simulink model "lab2_sliding_mode_control"  (R2018b)
settings: Solver=ode1  StartTime=0.0  StopTime=5  FixedStep=0.001  RelTol=1e-3  EnableMultiTasking=on
undefined symbols (not defined in the file or in its folder): HIL
libraries: quarc_library x5, simulink x1
settings Model: SimulationMode=external  ExtModeTrigDuration=100001  Creator=smascaro  LastModifiedBy=Student-No Password
settings SolverCC: PositivePriorityOrder=on
settings DataIOCC: LimitDataPoints=on  SaveFormat=Array  SignalLoggingSaveFormat=ModelDataLogs
settings OptimizationCC: ExpressionDepthLimit=2147483647  InitFltsAndDblsToZero=on  LifeSpan=inf
settings DebuggingCC: UnderspecifiedInitializationDetection=Classic  MergeDetectMultiDrivingBlocksExec=none  FcnCallInpInsideContextMsg=warning  AllowSymbolicDim=off  StateNameClashWarn=warning  SFUnexpectedBacktrackingDiag=warning  SFNoUnconditionalDefaultTransitionDiag=warning  SFExecutionAtInitializationDiag=none
settings HardwareCC: ProdBitPerPointer=32  ProdBitPerSizeT=32  ProdBitPerPtrDiffT=32  ProdLargestAtomicFloat=None  ProdIntDivRoundTo=Undefined  ProdEndianess=Unspecified  ProdWordSize=32  ProdHWDeviceType=32-bit Generic
settings ModelReferenceCC: PropagateSignalLabelsOutOfModel=off
settings SFSimCC: SimUseLocalCustomCode=off  SimParseCustomCode=off
settings RTWCC: SystemTargetFile=quarc_win64.tlc  TemplateMakefile=quarc_default_tmf  Description=QUARC Win64 Target  RTWUseLocalCustomCode=off
settings CodeAppCC: StateflowObjectComments=on
settings STFCustomTargetCC: TargetPreCompLibLocation=C:\PROGRA~3\QUARC\lib\2018b\win64\release  ConcurrentExecutionCompliant=on  GeneratePreprocessorConditionals=Disable all  CPPClassGenCompliant=on  GRTInterface=on  SystemTargetFile=quarc_win64.tlc
settings GRTTargetCC: TargetPreCompLibLocation=C:\PROGRA~3\QUARC\lib\2018b\win64\release  TargetLangStandard=C89/C90 (ANSI)  ParMdlRefBuildCompliant=off  CompOptLevelCompliant=off  GeneratePreprocessorConditionals=Disable all  CombineOutputUpdateFcns=off  MatFileLogging=off  GRTInterface=on  UseToolchainInfoCompliant=off  ExtMode=on  ExtModeMexFile=quarc_comm
settings ConfigComp: CovMetricSettings=dw  CovHtmlReporting=on  CovSaveCumulativeToWorkspaceVar=on  CovSaveSingleToWorkspaceVar=on  CovExternalEMLEnable=off

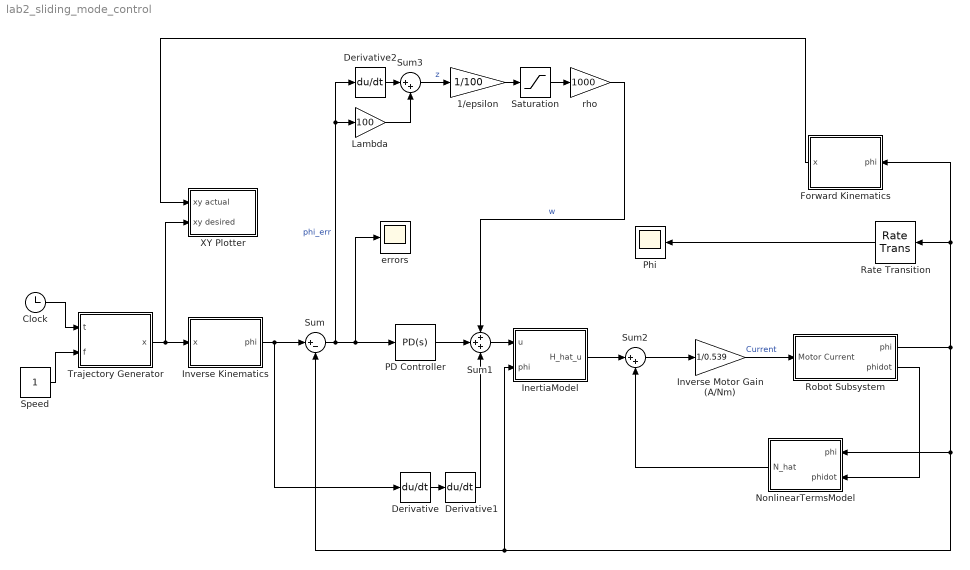
== system lab2_sliding_mode_control ==
  1/epsilon : Gain  Gain=1/100
  Clock : Clock
  Derivative : Derivative
  Derivative1 : Derivative
  Derivative2 : Derivative
  Forward Kinematics : MATLAB Function  TreatAsAtomicUnit=on
  InertiaModel : MATLAB Function  TreatAsAtomicUnit=on
  Inverse Kinematics : MATLAB Function  TreatAsAtomicUnit=on
  Inverse Motor Gain (A/Nm) : Gain  Gain=1/0.539
  Lambda : Gain  Gain=100
  NonlinearTermsModel : MATLAB Function  TreatAsAtomicUnit=on
  PD Controller : simulink/Continuous/PID Controller  Controller=PD  Form=Parallel  TimeDomain=Continuous-time  SampleTime=-1  IntegratorMethod=Forward Euler  FilterMethod=Forward Euler  ControllerParametersSource=internal  P=[1922;1922]  I=0  D=[40;40]  UseFilter=on  N=100  TunerSelectOption=Transfer Function Based (PID Tuner App)  InitialConditionSource=internal  InitialConditionForIntegrator=0  InitialConditionForFilter=0  DifferentiatorICPrevScaledInput=0  ExternalReset=none  TrackingMode=off  Kt=1  LimitOutput=off  UpperSaturationLimit=inf  LowerSaturationLimit=-inf  LinearizeAsGain=off  AntiWindupMode=none  Kb=1  POutMin=[]  POutMax=[]  IOutMin=[]  IOutMax=[]  DOutMin=[]  DOutMax=[]  NOutMin=[]  NOutMax=[]  SumOutMin=[]  SumOutMax=[]  SaturationOutMin=[]  SaturationOutMax=[]  PParamMin=[]  PParamMax=[]  IParamMin=[]  IParamMax=[]  DParamMin=[]  DParamMax=[]  NParamMin=[]  NParamMax=[]  KbParamMin=[]  KbParamMax=[]  KtParamMin=[]  KtParamMax=[]  KbOutMin=[]  KbOutMax=[]  KtOutMin=[]  KtOutMax=[]  IntegratorOutMin=[]  IntegratorOutMax=[]  FilterOutMin=[]  FilterOutMax=[]  SumI1OutMin=[]  SumI1OutMax=[]  SumI2OutMin=[]  SumI2OutMax=[]  SumI3OutMin=[]  SumI3OutMax=[]  SumI4OutMin=[]  SumI4OutMax=[]  SumDOutMin=[]  SumDOutMax=[]  DifferentiatorOutMin=[]  DifferentiatorOutMax=[]  FilterDiffOutCoefMin=[]  FilterDiffOutCoefMax=[]  ReciprocalOutMin=[]  ReciprocalOutMax=[]  SumDenOutMin=[]  SumDenOutMax=[]  SumNumOutMin=[]  SumNumOutMax=[]  DivideOutMin=[]  DivideOutMax=[]  IntegratorContinuousStateAttributes=''  IntegratorStateMustResolveToSignalObject=off  IntegratorRTWStateStorageClass=Auto  FilterContinuousStateAttributes=''  FilterStateMustResolveToSignalObject=off  FilterRTWStateStorageClass=Auto  ParallelPVariant=InternalParameters  IdealPVariant=Disabled  IVariant=Disabled  DVariant=InternalParameters  IntegratorVariant=Disabled  SatVariant=Disabled  AWVariant=Disabled  PCopyVariant=Disabled  TRVariant=Disabled  FdbkBlocksVariant=Forward  IdealPFdbkVariant=Disabled  SatFdbkVariant=Disabled  DerivativeFilterVariant=ContFilter  NVariant=InternalParameters  NCopyVariant=Disabled  FilterICVariant=InternalICsFilter  IntegratorICVariant=Disabled  ExternalResetVariant=Disabled  TRSumVariant=Passthrough  SumFdbkVariant=Disabled  SumVariant=Sum_PD
      settings: AttributesFormatString='PGain='%<P>\n'DGain='%<D>
  Phi : Scope
      settings: AttributesFormatString=SampleTime =%<SampleTime>
  Rate Transition : RateTransition  OutPortSampleTimeOpt=Inherit  OutPortSampleTimeMultiple=10  OutPortSampleTime=0.05
  Robot Subsystem : Subsystem
  Saturation : Saturate  UpperLimit=1  LowerLimit=-1
  Speed : Constant
      settings: AttributesFormatString=(circles/sec)
  Sum : Sum  Inputs=|+-
  Sum1 : Sum  Inputs=+++
  Sum2 : Sum  Inputs=|++
  Sum3 : Sum  Inputs=|++
  Trajectory Generator : MATLAB Function  TreatAsAtomicUnit=on
  XY Plotter : Subsystem
  errors : Scope
  rho : Gain  Gain=1000
  wires:
  Trajectory Generator/1(x) -> Inverse Kinematics/1(x), XY Plotter/2(xy desired)
  Clock/1 -> Trajectory Generator/1(t)
  Speed/1 -> Trajectory Generator/2(f)
  Forward Kinematics/1(x) -> XY Plotter/1(xy actual)
  PD Controller/1 -> Sum1/2
  Rate Transition/1 -> Phi/1
  Sum2/1 -> Inverse Motor Gain (A/Nm)/1
  InertiaModel/1(H_hat_u) -> Sum2/1
  Sum1/1 -> InertiaModel/1(u)
  Robot Subsystem/1(phi) -> Forward Kinematics/1(phi), Rate Transition/1, NonlinearTermsModel/1(phi), InertiaModel/2(phi), Sum/2
  Derivative/1 -> Derivative1/1
  Inverse Kinematics/1(phi) -> Derivative/1, Sum/1
  Derivative1/1 -> Sum1/3
  NonlinearTermsModel/1(N_hat) -> Sum2/2
  Inverse Motor Gain (A/Nm)/1 -> Robot Subsystem/1(Motor Current)  "Current"
  Robot Subsystem/2(phidot) -> NonlinearTermsModel/2(phidot)
  Sum3/1 -> 1/epsilon/1  "z"
  Saturation/1 -> rho/1
  Derivative2/1 -> Sum3/1
  Lambda/1 -> Sum3/2
  Sum/1 -> Lambda/1, Derivative2/1, errors/1, PD Controller/1  "phi_err"
  rho/1 -> Sum1/1  "w"
  1/epsilon/1 -> Saturation/1

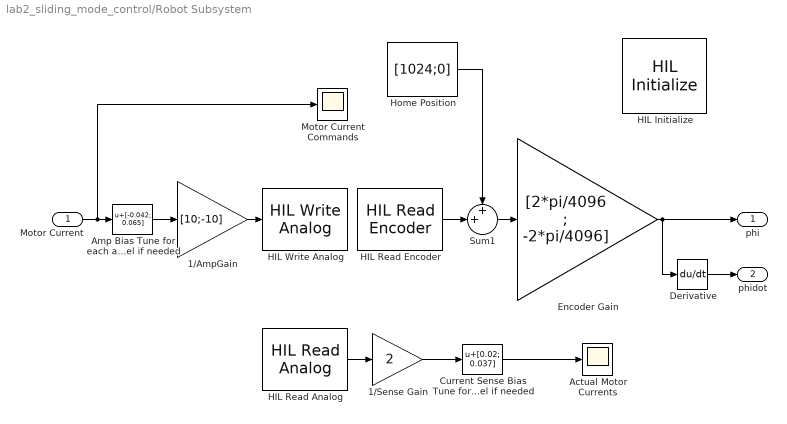
== system lab2_sliding_mode_control/Robot Subsystem ==
  Motor Current : Inport
  1/AmpGain : Gain  Gain=[10;-10]
  1/Sense Gain : Gain  Gain=2
  Actual Motor Currents : Scope
  Amp Bias Tune for each amp/channel if needed : Bias  Bias=[-0.042; 0.065]
  Current Sense Bias Tune for each amp/channel if needed : Bias  Bias=[0.02; 0.037]
  Derivative : Derivative
  Encoder Gain : Gain  Gain=[2*pi/4096 ; -2*pi/4096]
  HIL Initialize : quarc_library/Data Acquisition/Generic/Configuration/HIL Initialize  object_name=HIL-1  board_type=q8_usb  board_number=0  board_options=update_rate=normal  exclusive=off  active=off  hardware_clocks=[0:2]  clock_modes=[]  initial_clock_frequencies=[]  set_clock_params_at_start=off  set_clock_params_at_switch_in=off  set_clock_frequencies_at_start=off  set_clock_frequencies_at_switch_in=off  analog_input_channels=[0:7]  analog_input_configurations=[]  analog_input_maximums=10  analog_input_minimums=-10  set_analog_input_params_at_start=on  set_analog_input_params_at_switch_in=off  analog_output_channels=[0:7]  analog_output_maximums=10  analog_output_minimums=-10  initial_analog_outputs=[0]  final_analog_outputs=[0]  watchdog_analog_outputs=0  set_analog_output_params_at_start=on  set_analog_output_params_at_switch_in=off  set_analog_outputs_at_start=on  set_analog_outputs_at_switch_in=off  set_analog_outputs_at_terminate=on  set_analog_outputs_at_switch_out=off  set_analog_outputs_on_watchdog=off  digital_input_channels=[]  digital_output_channels=[]  digital_output_configuration=[]  initial_digital_outputs=[1]  final_digital_outputs=[1]  watchdog_digital_outputs=[1]  set_digital_output_params_at_start=off  set_digital_output_params_at_switch_in=off  set_digital_outputs_at_start=on  set_digital_outputs_at_switch_in=off  set_digital_outputs_at_terminate=on  set_digital_outputs_at_switch_out=off  set_digital_outputs_on_watchdog=off  encoder_channels=[0:7]  quadrature=[4]  encoder_filter_frequency=[]  initial_encoder_counts=[0]  set_encoder_params_at_start=on  set_encoder_params_at_switch_in=off  set_encoder_counts_at_start=on  set_encoder_counts_at_switch_in=off  pwm_channels=[0:7]  pwm_modes=0  pwm_frequency=99.532799999999995e6/4095  pwm_configuration=[0]  pwm_alignment=[0]  pwm_polarity=[1]  pwm_leading_deadband=[0]  pwm_trailing_deadband=[0]  initial_pwm_outputs=[0]  final_pwm_outputs=[0]  watchdog_pwm_outputs=[0]  set_pwm_params_at_start=on  set_pwm_params_at_switch_in=off  set_pwm_outputs_at_start=on  set_pwm_outputs_at_switch_in=off  set_pwm_outputs_at_terminate=on  set_pwm_outputs_at_switch_out=off  set_pwm_outputs_on_watchdog=off  other_output_channels=[]  initial_other_outputs=[]  final_other_outputs=[]  watchdog_other_outputs=[]  set_other_outputs_at_start=off  set_other_outputs_at_switch_in=off  set_other_outputs_at_terminate=off  set_other_outputs_at_switch_out=off  set_other_outputs_on_watchdog=off
  HIL Read Analog : quarc_library/Data Acquisition/Generic/Immediate I//O/HIL Read Analog  object_name=HIL-1  channels=[0;1]  sample_time=qc_get_step_size  active=on  vector_output=on
  HIL Read Encoder : quarc_library/Data Acquisition/Generic/Immediate I//O/HIL Read Encoder  object_name=HIL-1  channels=[0:1]  sample_time=qc_get_step_size  active=on  vector_output=on  data_type_mode=Inherit via back propagation  data_type=double
  HIL Write Analog : quarc_library/Data Acquisition/Generic/Immediate I//O/HIL Write Analog  object_name=HIL-1  channels=[0:1]  sample_time=-1  active=off  vector_input=on
  Home Position : Constant  Value=[1024;0]  VectorParams1D=off
  Motor Current Commands : Scope
  Sum1 : Sum  Inputs=++|
  phi : Outport
  phidot : Outport  Port=2
  wires:
  1/AmpGain/1 -> HIL Write Analog/1
  Encoder Gain/1 -> phi/1, Derivative/1
  Derivative/1 -> phidot/1
  HIL Read Analog/1 -> 1/Sense Gain/1
  Motor Current/1 -> Amp Bias Tune for each amp/channel if needed/1, Motor Current Commands/1
  Amp Bias Tune for each amp/channel if needed/1 -> 1/AmpGain/1
  Home Position/1 -> Sum1/1
  HIL Read Encoder/1 -> Sum1/2
  Sum1/1 -> Encoder Gain/1
  1/Sense Gain/1 -> Current Sense Bias Tune for each amp/channel if needed/1
  Current Sense Bias Tune for each amp/channel if needed/1 -> Actual Motor Currents/1

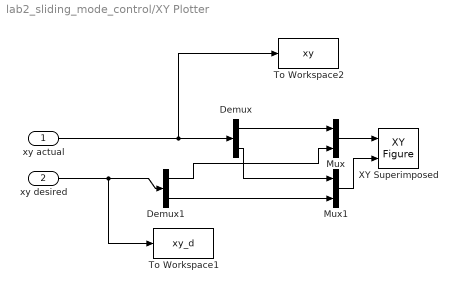
== system lab2_sliding_mode_control/XY Plotter ==
  xy actual : Inport
  xy desired : Inport  Port=2
  Demux : Demux  Outputs=2
  Demux1 : Demux  Outputs=2
  Mux : Mux  Inputs=2
  Mux1 : Mux  Inputs=2
  To Workspace1 : ToWorkspace  VariableName=xy_d  SampleTime=-1
  To Workspace2 : ToWorkspace  VariableName=xy  SampleTime=-1
  XY Superimposed : quarc_library/Sinks/Figures/XY Figure  figure_mode=Use figure window  figure_tag=figure1  axes_tag=axes1  minimum_x=0  maximum_x=.3  minimum_y=0  maximum_y=.2  buffer_size=10000  update_rate=100  initial_position="1033   623   623   411"  initial_visibility=off  sample_time=-1
      settings: SourceProductName=QUARC Targets
  wires:
  Demux/2 -> Mux1/1
  Mux1/1 -> XY Superimposed/2
  Mux/1 -> XY Superimposed/1
  Demux/1 -> Mux/1
  xy desired/1 -> Demux1/1, To Workspace1/1
  Demux1/1 -> Mux/2
  Demux1/2 -> Mux1/2
  xy actual/1 -> Demux/1, To Workspace2/1

== matlab function lab2_sliding_mode_control/Inverse Kinematics ==
  settings: fimath=|
      | fimath(...
      | 'RoundMode', 'floor',...
      | 'OverflowMode', 'wrap',...
      | 'ProductMode', 'KeepLSB', 'ProductWordLength', 32,...
      | 'SumMode', 'KeepLSB', 'SumWordLength', 32,...
      | 'CastBeforeSum', false)
  data: x input; phi output
function phi = fcn(x)
% This block supports an embeddable subset of the MATLAB language.
% See the help menu for details. 
a1=0.15;
a2=0.15;
Jt = [1 0; -1 1]; % belt drive Jabobian
theta = [0;0];
theta(2) = -2*atan(sqrt(((a1+a2)^2-(x(1)^2+x(2)^2))/((x(1)^2+x(2)^2)-(a1-a2)^2)));
theta(1) = atan2(x(2),x(1))-atan2(a2*sin(theta(2)),a1+a2*cos(theta(2)));
phi = inv(Jt)*theta; % convert to absolute joint angles

== matlab function lab2_sliding_mode_control/Forward Kinematics ==
  settings: fimath=|
      | fimath(...
      | 'RoundMode', 'floor',...
      | 'OverflowMode', 'wrap',...
      | 'ProductMode', 'KeepLSB', 'ProductWordLength', 32,...
      | 'SumMode', 'KeepLSB', 'SumWordLength', 32,...
      | 'CastBeforeSum', false)
  data: x output; phi input
function x = fcn(phi)
% This block supports an embeddable subset of the MATLAB language.
% See the help menu for details. 
a1=.15;
a2=.15;
x = [0;0];
x(1) = a1*cos(phi(1))+a2*cos(phi(2));
x(2) = a1*sin(phi(1))+a2*sin(phi(2));

== matlab function lab2_sliding_mode_control/InertiaModel ==
  settings: fimath=|
      | fimath(...
      | 'RoundMode', 'floor',...
      | 'OverflowMode', 'wrap',...
      | 'ProductMode', 'KeepLSB', 'ProductWordLength', 32,...
      | 'SumMode', 'KeepLSB', 'SumWordLength', 32,...
      | 'CastBeforeSum', false)
  data: u input double size=2; phi input double size=2; H_hat_u output double size=2
function H_hat_u = fcn(u,phi)
% This block supports an embeddable subset of the MATLAB language.
% See the help menu for details. 

a1 = 0.15;  % link 1 length
a2 = 0.15;  % link 2 length
m1 = 0.092;  % link 1 mass  
m2 = 0.077; % link 2 mas
r01 = 0.062; % link 1 center of mass
r12 = 0.036; % link 2 COM
I1 = 0.64e-3;  % link 1 inertia
I2 = 0.30e-3;  % link 2 inertia
Jm1 = 0.65e-6; % motor inertias
Jm2 = 0.65e-6;
b1 = 3.1e-6; % viscous damping constants
b2 = 3.1e-6;
c1 = 0.0001; % coulomb friction constants
c2 = 0.0001;
g = 9.8; % gravitational constant
N1 = 70; % gear ratios
N2 = 70;

H11 = N1^2*Jm1 + I1 + m2*a1^2;
H12 = a1*r12*m2*cos(phi(2)-phi(1));
H21 = H12;
H22 = N2^2*Jm2 + I2;

H_hat = [H11 H12; H21 H22]; % inertia matrix

H_hat_u = H_hat*u;

== matlab function lab2_sliding_mode_control/NonlinearTermsModel ==
  settings: fimath=|
      | fimath(...
      | 'RoundMode', 'floor',...
      | 'OverflowMode', 'wrap',...
      | 'ProductMode', 'KeepLSB', 'ProductWordLength', 32,...
      | 'SumMode', 'KeepLSB', 'SumWordLength', 32,...
      | 'CastBeforeSum', false)
  data: phi input double size=2; phidot input double size=2; N_hat output double size=2
function N_hat = fcn(phi,phidot)
% This block supports an embeddable subset of the MATLAB language.
% See the help menu for details. 

a1 = 0.15;  % link 1 length
a2 = 0.15;  % link 2 length
m1 = 0.092;  % link 1 mass  
m2 = 0.077; % link 2 mas
r01 = 0.062; % link 1 center of mass
r12 = 0.036; % link 2 COM
I1 = 0.64e-3;  % link 1 inertia
I2 = 0.30e-3;  % link 2 inertia
Jm1 = 0.65e-6; % motor inertias
Jm2 = 0.65e-6;
b1 = 3.1e-6; % viscous damping constants
b2 = 3.1e-6;
c1 = 0.0001; % coulomb friction constants
c2 = 0.0001;
g = 9.8; % gravitational constant
N1 = 70; % gear ratios
N2 = 70;

h = a1*r12*m2*sin(phi(2)-phi(1));
G1 = (r01*m1+a1*m2)*g*cos(phi(1));
G2 = r12*m2*g*cos(phi(2));
F1 = N1^2*b1*phidot(1) + N1*c1*sign(phidot(1));
F2 = N2^2*b2*phidot(2) + N2*c2*sign(phidot(2));

V_hat = [0 -h ;h 0]*[phidot(1)^2;phidot(2)^2]; % centripetal torques
G_hat = [G1;G2]; % gravity torques
F_hat = [F1;F2]; % frictional torques

N_hat = V_hat + G_hat + F_hat;

== matlab function lab2_sliding_mode_control/Trajectory Generator ==
  settings: fimath=|
      | fimath(...
      | 'RoundMode', 'floor',...
      | 'OverflowMode', 'wrap',...
      | 'ProductMode', 'KeepLSB', 'ProductWordLength', 32,...
      | 'SumMode', 'KeepLSB', 'SumWordLength', 32,...
      | 'CastBeforeSum', false)
  data: x output; t input; f input
function x = fcn(t,f)
% This block supports an embeddable subset of the MATLAB language.
% See the help menu for details. 
x = [0;0];

if t<1 % move robot smoothly from home position @ x=[1.5,1.5] to point on circle @ x=[0.2,0.1]
        x(1) = 0.15 + 0.025*(1 - cos(pi*t));
        x(2) = 0.15 - 0.025*(1 - cos(pi*t));
elseif t<1.5  % accelerate into circling trajectory
    x(1) = 0.075*cos(2*pi*f*(t-1)^2) + 0.125;
    x(2) = 0.075*sin(2*pi*f*(t-1)^2) + 0.1;
else  % constant speed circling of radius 0.075 about x=[0.125,0.1]
    x(1) = 0.075*cos(2*pi*f*(t-1.25)) + 0.125;
    x(2) = 0.075*sin(2*pi*f*(t-1.25)) + 0.1;
end
